simulink model "Mux_Demux"  (R2018b)
settings: Solver=VariableStepAuto  StartTime=0.0  StopTime=10.0  RelTol=1e-3
settings Model: Creator=domin  LastModifiedBy=domin

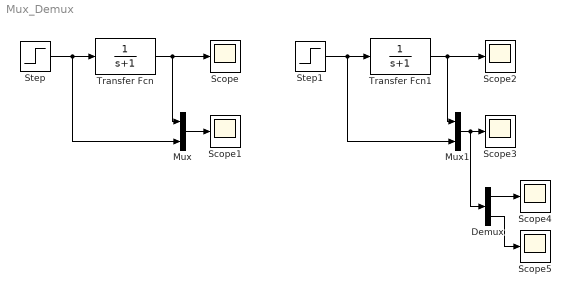
== system Mux_Demux ==
  Demux : Demux  Outputs=2
  Mux : Mux  Inputs=2
  Mux1 : Mux  Inputs=2
  Scope{,1..5} (6 alike) : Scope
  Step : Step  SampleTime=0
  Step1 : Step  SampleTime=0
  Transfer Fcn : TransferFcn  Denominator=[1 1]
  Transfer Fcn1 : TransferFcn  Denominator=[1 1]
  wires:
  Step/1 -> Mux/2, Transfer Fcn/1
  Transfer Fcn/1 -> Mux/1, Scope/1
  Mux/1 -> Scope1/1
  Mux1/1 -> Demux/1, Scope3/1
  Transfer Fcn1/1 -> Mux1/1, Scope2/1
  Step1/1 -> Mux1/2, Transfer Fcn1/1
  Demux/1 -> Scope4/1
  Demux/2 -> Scope5/1
